simulink model "PC_Quadcopter_Simulation_online_learning"  (R2017a)
settings: Solver=ode45  StartTime=0.0  StopTime=20  FixedStep=0.05  MaxStep=0.06  RelTol=1e-3  EnableMultiTasking=on
model workspace (MAT data in the model file):
  MCOS : class17 (value not decoded)
undefined symbols (not defined in the file or in its folder): error1, error2, error3, error4, IC, quadModel
libraries: simulink x4
(part 2 of 2)

== system PC_Quadcopter_Simulation_online_learning/Quadcopter Dynamics/External Disturbances ==
  note: Note: Torques are in units of N*m, Forces in N
      | Torques are applied to the BODY coordinate system.
      | Forces are applied from the WORLD coordinate system!
      | This can be changed by adjusting the equations within the S-function.
  Bus Creator : BusCreator  Inputs=6
  Bus to Vector : BusToVector
  Constant{2..6} (5 alike) : Constant  Value=0
  Step : Step  After=0  SampleTime=0
  "Disturbances " : Outport
  wires:
  Bus to Vector/1 -> "Disturbances "/1
  Bus Creator/1 -> Bus to Vector/1
  Constant6/1 -> Bus Creator/1  "Tau_bx-axis"
  Step/1 -> Bus Creator/2  "Tau_by-axis"
  Constant2/1 -> Bus Creator/3  "Tau_bz-axis"
  Constant3/1 -> Bus Creator/4  "Force_x-axis"
  Constant4/1 -> Bus Creator/5  "Force_y-axis"
  Constant5/1 -> Bus Creator/6  "Force_z-axis"

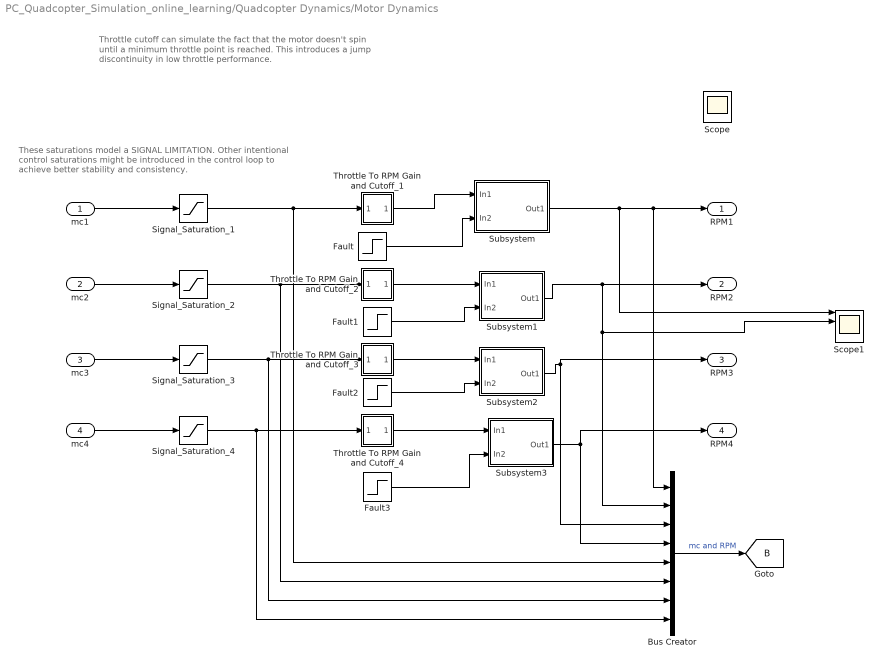
== system PC_Quadcopter_Simulation_online_learning/Quadcopter Dynamics/Motor Dynamics ==
  note: Throttle cutoff can simulate the fact that the motor doesn't
      | spin until a minimum throttle point is reached. This introduces
      | a jump discontinuity in low throttle performance.
  note: These saturations model a SIGNAL LIMITATION.
      | Other intentional control saturations might be introduced in the
      | control loop to achieve better stability and consistency.
  mc1 : Inport
  mc2 : Inport  Port=2
  mc3 : Inport  Port=3
  mc4 : Inport  Port=4
  Bus Creator : BusCreator  Inputs=8
  Fault : Step  Time=15  After=error1  SampleTime=0
  Fault1 : Step  Time=15  After=error2  SampleTime=0
  Fault2 : Step  Time=15  After=error3  SampleTime=0
  Fault3 : Step  Time=15  After=error4  SampleTime=0
  Scope : Scope  NumInputPorts=2
  Scope1 : Scope  NumInputPorts=4
  Signal_Saturation_{1..4} (4 alike) : Saturate  UpperLimit=100  LowerLimit=0
  Subsystem : Subsystem
  Subsystem1 : Subsystem
  Subsystem2 : Subsystem
  Subsystem3 : Subsystem
  Throttle To RPM Gain and Cutoff_1 : Subsystem
  Throttle To RPM Gain and Cutoff_2 : Subsystem
  Throttle To RPM Gain and Cutoff_3 : Subsystem
  Throttle To RPM Gain and Cutoff_4 : Subsystem
  RPM1 : Outport
  RPM2 : Outport  Port=2
  RPM3 : Outport  Port=3
  RPM4 : Outport  Port=4
  tag scope: B=global
  wires:
  mc1/1 -> Signal_Saturation_1/1
  mc4/1 -> Signal_Saturation_4/1
  mc2/1 -> Signal_Saturation_2/1
  mc3/1 -> Signal_Saturation_3/1
  Signal_Saturation_1/1 -> Bus Creator/5, Throttle To RPM Gain and Cutoff_1/1(In5)
  Signal_Saturation_2/1 -> Bus Creator/6, Throttle To RPM Gain and Cutoff_2/1(In5)
  Signal_Saturation_3/1 -> Bus Creator/7, Throttle To RPM Gain and Cutoff_3/1(In5)
  Signal_Saturation_4/1 -> Bus Creator/8, Throttle To RPM Gain and Cutoff_4/1(In5)
  Throttle To RPM Gain and Cutoff_4/1(Out5) -> Subsystem3/1(In1)
  Subsystem3/1(Out1) -> RPM4/1, Bus Creator/4
  Bus Creator/1 -> [B]  "mc and RPM"
  Subsystem/1(Out1) -> Scope1/1, Bus Creator/1, RPM1/1
  Throttle To RPM Gain and Cutoff_1/1(Out5) -> Subsystem/1(In1)
  Fault/1 -> Subsystem/2(In2)
  Subsystem2/1(Out1) -> Bus Creator/3, RPM3/1
  Subsystem1/1(Out1) -> Scope1/2, Bus Creator/2, RPM2/1
  Throttle To RPM Gain and Cutoff_2/1(Out5) -> Subsystem1/1(In1)
  Throttle To RPM Gain and Cutoff_3/1(Out5) -> Subsystem2/1(In1)
  Fault2/1 -> Subsystem2/2(In2)
  Fault3/1 -> Subsystem3/2(In2)
  Fault1/1 -> Subsystem1/2(In2)

== system PC_Quadcopter_Simulation_online_learning/Quadcopter Dynamics/Motor Dynamics/Subsystem ==
  In1 : Inport
  In2 : Inport  Port=2
  MATLAB Function : MATLAB Function  TreatAsAtomicUnit=on
  Motor_Dynamics_1 : StateSpace  A=-1/quadModel.T  C=1/quadModel.T  D=0  X0=IC.w1*quadModel.T
  Scope : Scope  NumInputPorts=4
  Out1 : Outport
  wires:
  In1/1 -> Motor_Dynamics_1/1
  MATLAB Function/1(rotor_speed) -> Scope/3, Out1/1
  In2/1 -> MATLAB Function/1(fault)
  Motor_Dynamics_1/1 -> Scope/2, MATLAB Function/2(nominal_model_input)

== system PC_Quadcopter_Simulation_online_learning/Quadcopter Dynamics/Motor Dynamics/Subsystem1 ==
  In1 : Inport
  In2 : Inport  Port=2
  MATLAB Function : MATLAB Function  TreatAsAtomicUnit=on
  "Motor_Dynamics_2 " : StateSpace  A=-1/quadModel.T  C=1/quadModel.T  D=0  X0=IC.w1*quadModel.T
  Out1 : Outport
  wires:
  In1/1 -> "Motor_Dynamics_2 "/1
  MATLAB Function/1(rotor_speed) -> Out1/1
  In2/1 -> MATLAB Function/1(fault)
  "Motor_Dynamics_2 "/1 -> MATLAB Function/2(nominal_modal_input)

== system PC_Quadcopter_Simulation_online_learning/Quadcopter Dynamics/Motor Dynamics/Subsystem2 ==
  In1 : Inport
  In2 : Inport  Port=2
  MATLAB Function : MATLAB Function  TreatAsAtomicUnit=on
  "Motor_Dynamics_3 " : StateSpace  A=-1/quadModel.T  C=1/quadModel.T  D=0  X0=IC.w1*quadModel.T
  Out1 : Outport
  wires:
  In1/1 -> "Motor_Dynamics_3 "/1
  MATLAB Function/1(rotor_speed) -> Out1/1
  In2/1 -> MATLAB Function/1(fault)
  "Motor_Dynamics_3 "/1 -> MATLAB Function/2(nominal_modal_input)

== system PC_Quadcopter_Simulation_online_learning/Quadcopter Dynamics/Motor Dynamics/Subsystem3 ==
  In1 : Inport
  In2 : Inport  Port=2
  MATLAB Function : MATLAB Function  TreatAsAtomicUnit=on
  "Motor_Dynamics_4 " : StateSpace  A=-1/quadModel.T  C=1/quadModel.T  D=0  X0=IC.w1*quadModel.T
  Out1 : Outport
  wires:
  In1/1 -> "Motor_Dynamics_4 "/1
  MATLAB Function/1(rotor_speed) -> Out1/1
  In2/1 -> MATLAB Function/1(fault)
  "Motor_Dynamics_4 "/1 -> MATLAB Function/2(nominal_modal_input)

== system PC_Quadcopter_Simulation_online_learning/Quadcopter Dynamics/Motor Dynamics/Throttle To RPM Gain and Cutoff_1 ==
  note: minThr should be a quad.mat value
  note: This gain should be a quad.mat value
  note: This constant should be a quad.mat value
  note: Output equals linearly scaled RPM
      | for given throttle input if throttle input >=Throttle Cuttoff (minThr)
      | else output is zero.
  In5 : Inport
  Constant : Constant  Value=quadModel.b
  Gain : Gain  Gain=quadModel.cr
  Minimum Throttle Cutoff : simulink/Logic and Bit Operations/Compare To Constant  relop=>=  const=quadModel.minThr  OutDataTypeStr=uint8
  Product : Product
  Sum1 : Sum  Inputs=++|
  Out5 : Outport
  wires:
  Minimum Throttle Cutoff/1 -> Product/2
  Product/1 -> Out5/1
  In5/1 -> Gain/1, Minimum Throttle Cutoff/1
  Gain/1 -> Sum1/2
  Sum1/1 -> Product/1
  Constant/1 -> Sum1/1

== system PC_Quadcopter_Simulation_online_learning/Quadcopter Dynamics/Motor Dynamics/Throttle To RPM Gain and Cutoff_2 ==
  note: minThr should be a quad.mat value
  note: This gain should be a quad.mat value
  note: This constant should be a quad.mat value
  note: Output equals linearly scaled RPM
      | for given throttle input if throttle input >=Throttle Cuttoff (minThr)
      | else output is zero.
  In5 : Inport
  Constant : Constant  Value=quadModel.b
  Gain : Gain  Gain=quadModel.cr
  Minimum Throttle Cutoff : simulink/Logic and Bit Operations/Compare To Constant  relop=>=  const=quadModel.minThr  OutDataTypeStr=uint8
  Product : Product
  Sum1 : Sum  Inputs=++|
  Out5 : Outport
  wires:
  Minimum Throttle Cutoff/1 -> Product/2
  Product/1 -> Out5/1
  In5/1 -> Gain/1, Minimum Throttle Cutoff/1
  Gain/1 -> Sum1/2
  Sum1/1 -> Product/1
  Constant/1 -> Sum1/1

== system PC_Quadcopter_Simulation_online_learning/Quadcopter Dynamics/Motor Dynamics/Throttle To RPM Gain and Cutoff_3 ==
  note: minThr should be a quad.mat value
  note: This gain should be a quad.mat value
  note: This constant should be a quad.mat value
  note: Output equals linearly scaled RPM
      | for given throttle input if throttle input >=Throttle Cuttoff (minThr)
      | else output is zero.
  In5 : Inport
  Constant : Constant  Value=quadModel.b
  Gain : Gain  Gain=quadModel.cr
  Minimum Throttle Cutoff : simulink/Logic and Bit Operations/Compare To Constant  relop=>=  const=quadModel.minThr  OutDataTypeStr=uint8
  Product : Product
  Sum1 : Sum  Inputs=++|
  Out5 : Outport
  wires:
  Minimum Throttle Cutoff/1 -> Product/2
  Product/1 -> Out5/1
  In5/1 -> Gain/1, Minimum Throttle Cutoff/1
  Gain/1 -> Sum1/2
  Sum1/1 -> Product/1
  Constant/1 -> Sum1/1

== system PC_Quadcopter_Simulation_online_learning/Quadcopter Dynamics/Motor Dynamics/Throttle To RPM Gain and Cutoff_4 ==
  note: minThr should be a quad.mat value
  note: This gain should be a quad.mat value
  note: This constant should be a quad.mat value
  note: Output equals linearly scaled RPM
      | for given throttle input if throttle input >=Throttle Cuttoff (minThr)
      | else output is zero.
  In5 : Inport
  Constant : Constant  Value=quadModel.b
  Gain : Gain  Gain=quadModel.cr
  Minimum Throttle Cutoff : simulink/Logic and Bit Operations/Compare To Constant  relop=>=  const=quadModel.minThr  OutDataTypeStr=uint8
  Product : Product
  Sum1 : Sum  Inputs=++|
  Out5 : Outport
  wires:
  Minimum Throttle Cutoff/1 -> Product/2
  Product/1 -> Out5/1
  In5/1 -> Gain/1, Minimum Throttle Cutoff/1
  Gain/1 -> Sum1/2
  Sum1/1 -> Product/1
  Constant/1 -> Sum1/1

== matlab function PC_Quadcopter_Simulation_online_learning/Quadcopter Dynamics/Motor Dynamics/Subsystem/MATLAB Function ==
  data: fault input; nominal_model_input input; rotor_speed output
function rotor_speed = fcn(fault, nominal_model_input)

rotor_speed =(nominal_model_input* (1-fault));

end

== matlab function PC_Quadcopter_Simulation_online_learning/Attitude Controller/blending  ==
  data: control_signal output; portion input; fault_controller input; nominal_controller input
function control_signal = blending(portion , fault_controller, nominal_controller)

fault_part = (fault_controller * portion);
nominal_portion = 1-portion;
nominal_part = nominal_controller * nominal_portion;
control_signal = fault_part + nominal_part;

end

== matlab function PC_Quadcopter_Simulation_online_learning/Quadcopter Dynamics/Motor Dynamics/Subsystem1/MATLAB Function ==
  data: fault input; nominal_modal_input input; rotor_speed output
function rotor_speed = fcn(  fault, nominal_modal_input)


rotor_speed =  (nominal_modal_input* (1-fault));

end

== matlab function PC_Quadcopter_Simulation_online_learning/Position Controller/MATLAB Function ==
  data: y_error input; x_error input; max_error_signal data_store_memory
function fcn(y_error,x_error)

global max_error_signal;

%if(abs(y_error) + abs(x_error) > max_error_signal)
max_error_signal = max_error_signal + abs(y_error) + abs(x_error);

end

== matlab function PC_Quadcopter_Simulation_online_learning/Quadcopter Dynamics/Motor Dynamics/Subsystem2/MATLAB Function ==
  data: fault input; nominal_modal_input input; rotor_speed output
function rotor_speed = fcn(  fault, nominal_modal_input)


rotor_speed =  (nominal_modal_input* (1-fault));

end

== matlab function PC_Quadcopter_Simulation_online_learning/Quadcopter Dynamics/Motor Dynamics/Subsystem3/MATLAB Function ==
  data: fault input; nominal_modal_input input; rotor_speed output
function rotor_speed = fcn(  fault, nominal_modal_input)


rotor_speed =  (nominal_modal_input* (1-fault));

end

== matlab function PC_Quadcopter_Simulation_online_learning/Attitude Controller/blending 1 ==
  data: control_signal output; portion input; fault_controller input; nominal_controller input
function control_signal = blending(portion , fault_controller, nominal_controller)

fault_part = (fault_controller * portion);
nominal_portion = 1-portion;
nominal_part = nominal_controller * nominal_portion;
control_signal = fault_part + nominal_part;

end

== matlab function PC_Quadcopter_Simulation_online_learning/Attitude Controller/blending 2 ==
  data: control_signal output; portion input; fault_controller input; nominal_controller input
function control_signal = blending(portion , fault_controller, nominal_controller)

fault_part = (fault_controller * portion);
nominal_portion = 1-portion;
nominal_part = nominal_controller * nominal_portion;
control_signal = fault_part + nominal_part;

end

== matlab function PC_Quadcopter_Simulation_online_learning/Attitude Controller/High level Controller /MATLAB Function1 ==
  data: done input; BlendOne output; BlendTwo output; BlendThree output
function [BlendOne, BlendTwo, BlendThree]= fcn(done)


    BlendOne = rand();
    BlendTwo = rand();
    BlendThree = rand();

== matlab function PC_Quadcopter_Simulation_online_learning/Attitude Controller/High level Controller /MATLAB Function2 ==
  data: error1 input; Phi output; error2 input; error3 input; blend1 input; blend2 input; blend3 input; Theta output; Psi output
function [Phi, Theta , Psi] = fcn(error1, error2, error3, blend1, blend2, blend3)
errors = [error1, error2, error3];
min_errors = min(errors);

switch min_errors
    case error1
        Phi = blend1;
        Theta = blend1;
        Psi = blend1;
    case error2
        Phi = blend2;
        Theta = blend2;
        Psi = blend2;
    otherwise
        Phi = blend3;
        Theta = blend3;
        Psi = blend3;
end

== matlab function PC_Quadcopter_Simulation_online_learning/Attitude Controller/High level Controller /MATLAB Function ==
  data: r1 input; done output; r2 input; r3 input; r4 input; X input; Y input; Psi input; U input; V input; Phi input; W input; P input; The input; Q input; R input; Z input; time input; previousTime data_store_memory; sim_error data_store_memory; sim_iteration data_store_memory; result data_store_memory; Phi_blend data_store_memory; Psi_blend data_store_memory; Theta_blend data_store_memory; r1_speed input; r2_speed input; r3_speed input; r4_speed input; sig_5 input; sig_6 input; sig_8 input; sig_7 input; Phi_Cmd input; The_Cmd input; Psi_Cmd input; Alt_Cmd input; X_Cmd input; Y_Cmd input; sim_state_X data_store_memory; sim_state_Y data_store_memory; sim_state_Z data_store_memory; sim_state_U data_store_memory; sim_state_V data_store_memory; sim_state_W data_store_memory; sim_state_P data_store_memory; sim_state_Q data_store_memory; sim_state_R data_store_memory; sim_state_Phi data_store_memory; sim_state_The data_store_memory; sim_state_Psi data_store_memory; sim_state_r1_speed data_store_memory; sim_state_r2_speed data_store_memory; sim_state_r3_speed data_store_memory; sim_state_r4_speed data_store_memory; sim_state_sig_5 data_store_memory; sim_state_sig_6 data_store_memory; sim_state_sig_7 data_store_memory; sim_state_sig_8 data_store_memory; sim_state_Phi_Cmd data_store_memory; sim_state_The_Cmd data_store_memory; sim_state_Psi_Cmd data_store_memory; sim_state_Alt_Cmd data_store_memory; sim_state_X_Cmd data_store_memory; sim_state_Y_Cmd data_store_memory; error1 data_store_memory; error2 data_store_memory; error3 data_store_memory; error4 data_store_memory; Phi_sim_blend data_store_memory; Theta_sim_blend data_store_memory; Psi_sim_blend data_store_memory
function done     = fcn(r1, r2 , r3, r4 ,X, Y, Psi , U , V, Phi,    W,  P , The, Q , R, Z, time , r1_speed ,r2_speed,r3_speed,r4_speed, sig_5 , sig_6, sig_8, sig_7 , Phi_Cmd, The_Cmd, Psi_Cmd, Alt_Cmd, X_Cmd, Y_Cmd)
%coder.extrinsic('sim');
coder.extrinsic('run');
coder.extrinsic('assignin');
coder.extrinsic('struct');
coder.extrinsic('evalin');
global previousTime;

%global sim_error;
%global sim_iteration;
%global result;
%global Phi_blend;
%global Theta_blend;
%global Psi_blend;

global sim_state_P;
global sim_state_R;
global sim_state_Phi;
global sim_state_The;
global sim_state_Psi;
global sim_state_U;
global sim_state_Q;
global sim_state_V;
global sim_state_W;
global sim_state_X;
global sim_state_Y;
global sim_state_Z;
global sim_state_r1_speed;
global sim_state_r2_speed;
global sim_state_r3_speed;
global sim_state_r4_speed;
global sim_state_sig_5;
global sim_state_sig_6;
global sim_state_sig_7;
global sim_state_sig_8;
global sim_state_Phi_Cmd;
global sim_state_The_Cmd;
global sim_state_Psi_Cmd;
global sim_state_Alt_Cmd;
global sim_state_X_Cmd;
global sim_state_Y_Cmd;

%global Phi_sim_blend;
%global Theta_sim_blend;
%global Psi_sim_blend;


sim_time = 2;

if(previousTime+1 < time)
    
    previousTime = int16(time);
    
    %  n = 3;
    
    % result = zeros(1,n);
    %Phi_blend = zeros(1,n);
    %Theta_blend = zeros(1,n);
    %Psi_blend = zeros(1,n);
    
    X_goal = X+sim_time;
    X_t = [ X, X_goal]; % meters
    Y_t = [ Y, 0]; % meters
    Z_t = [ Z, 3]; % meters
    t = [ 0, sim_time]; % seconds
    Psi_t = [Psi, 0]; % radians
    
    assignin('base', 'X_t', X_t)
    assignin('base', 'Y_t', Y_t)
    assignin('base', 'Z_t', Z_t)
    assignin('base', 't', t)
    assignin('base', 'Psi_t', Psi_t)
    
    run('generate_sim_path');
    %for i = 1:n
    %{
        sim_state_values = struct('X' , X , 'Y',Y, 'Psi', Psi , 'U', U, 'V', V, 'Phi', Phi, 'P', P, 'The', The, 'Q',  Q, 'W', W, 'R', R, 'Z', Z, 'r1_speed', r1_speed, 'r2_speed', r2_speed , 'r3_speed', r3_speed, 'r4_speed', r4_speed, 'sig_5',  sig_5 , 'sig_6' , sig_6 , 'sig_7' ,sig_7, 'sig_8', sig_8, 'Phi_Cmd', Phi_Cmd, 'The_Cmd', The_Cmd, 'Psi_Cmd', Psi_Cmd, 'Alt_Cmd', Alt_Cmd, 'X_Cmd', X_Cmd, 'Y_Cmd', Y_Cmd );
        sim_state_lables = 'blah';
        sim_state = struct('values', sim_state_values, 'label', sim_state_lables, 'blockName' , 'placeholder');
        
        disp(sim_state);
        assignin('base', 'sim_state',sim_state );
    %}
    sim_state_X = X;
    sim_state_Y = Y;
    sim_state_Psi = Psi;
    sim_state_U = U;
    sim_state_V = V;
    sim_state_Phi = Phi;
    sim_state_P = P;
    sim_state_The = The;
    sim_state_Q = Q;
    sim_state_W = W;
    sim_state_R = R;
    sim_state_Z = Z;
    sim_state_r1_speed = r1_speed ;
    sim_state_r2_speed = r2_speed;
    sim_state_r3_speed = r3_speed;
    sim_state_r4_speed =r4_speed;
    sim_state_sig_5 = sig_5;
    sim_state_sig_6 = sig_6;
    sim_state_sig_8 = sig_8;
    sim_state_sig_7 = sig_7;
    sim_state_Phi_Cmd =  Phi_Cmd;
    sim_state_The_Cmd = The_Cmd;
    sim_state_Psi_Cmd= Psi_Cmd;
    sim_state_Alt_Cmd = Alt_Cmd;
    sim_state_X_Cmd = X_Cmd;
    sim_state_Y_Cmd = Y_Cmd;
    
    
    assignin('base', 'sim_state_X',sim_state_X );
    assignin('base', 'sim_state_Y',sim_state_Y );
    assignin('base', 'sim_state_Psi',sim_state_Psi );
    assignin('base', 'sim_state_U',sim_state_U );
    assignin('base', 'sim_state_V',sim_state_V );
    assignin('base', 'sim_state_Phi', sim_state_Phi);
    assignin('base', 'sim_state_P',sim_state_P );
    assignin('base', 'sim_state_The',sim_state_The );
    assignin('base', 'sim_state_Q', sim_state_Q);
    assignin('base', 'sim_state_W',sim_state_W );
    assignin('base', 'sim_state_R', sim_state_R);
    assignin('base', 'sim_state_Z', sim_state_Z);
    assignin('base', 'sim_state_r1_speed', sim_state_r1_speed);
    assignin('base', 'sim_state_r2_speed', sim_state_r2_speed);
    assignin('base', 'sim_state_r3_speed', sim_state_r3_speed);
    assignin('base', 'sim_state_r4_speed', sim_state_r4_speed);
    assignin('base', 'sim_state_sig_5', sim_state_sig_5);
    assignin('base', 'sim_state_sig_8',sim_state_sig_8 );
    assignin('base', 'sim_state_sig_7', sim_state_sig_7);
    assignin('base', 'sim_state_sig_6', sim_state_sig_6);
    assignin('base', 'sim_state_Phi_Cmd', sim_state_Phi_Cmd);
    assignin('base', 'sim_state_The_Cmd', sim_state_The_Cmd);
    assignin('base', 'sim_state_Psi_Cmd', sim_state_Psi_Cmd);
    assignin('base', 'sim_state_Alt_Cmd', sim_state_Alt_Cmd);
    assignin('base', 'sim_state_X_Cmd', sim_state_X_Cmd);
    assignin('base', 'sim_state_Y_Cmd',sim_state_Y_Cmd );
    
    
    %res = run('run_partial_simulation');
    %disp(res);
    %record sim result
    
    %disp(Phi_sim_blend);
    %disp(Theta_sim_blend);
    %disp(Psi_sim_blend);
    % result(n) = sim_error;
    % Phi_blend(n) = Phi_sim_blend;
    % Theta_blend(n) = Theta_sim_blend;
    % Psi_blend(n) = Psi_sim_blend ;
    
    
    done = 1;
else
    done = 0;
end

%update Q matrices
%end

%output next step for
%[ val , index ] = min(result);
%Psi = Phi_blend(index);
%Theta = Theta_blend(index);
%Phi = Phi_blend(index);
